simulink model "DFNN_EFS"  (R2022a)
settings: Solver=ode1  StartTime=0.0  StopTime=4*pi  FixedStep=0.001  RelTol=1e-3
libraries: roblocks x1
settings Model: Creator=DELL  LastModifiedBy=qinyi
settings DebuggingCC: UnconnectedInputMsg=warning  UnconnectedOutputMsg=warning  UnconnectedLineMsg=warning
settings RTWCC: DLArmComputeVersion=19.05

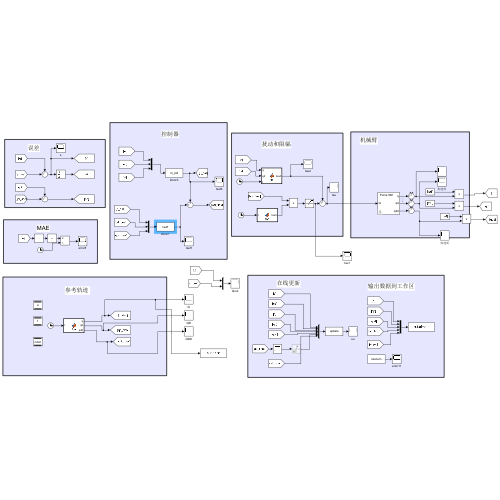
[thumbnail: Simulink's stored preview of the top-level diagram]
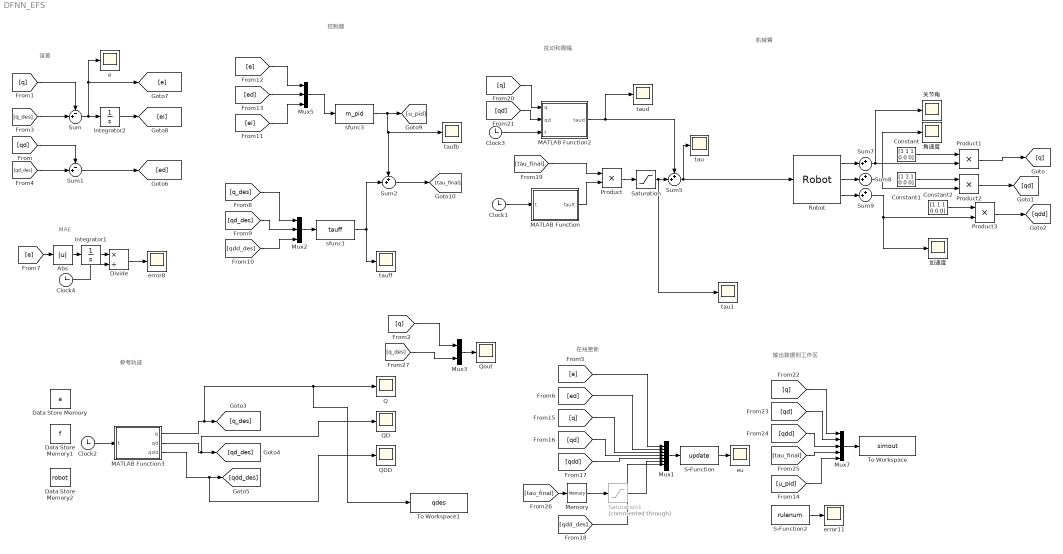
== system DFNN_EFS ==
  note: 在线更新
  note: MAE
  note: 机械臂
  note: 扰动和限幅
  note: 控制器
  note: 误差
  note: 参考轨迹
  note: 输出数据到工作区
  Abs : Abs  SaturateOnIntegerOverflow=off
  Clock{1..4} (4 alike) : Clock
  Constant : Constant  Value=[1 1 1 0 0 0]
  Constant1 : Constant  Value=[1 1 1 0 0 0]
  Constant2 : Constant  Value=[1 1 1 0 0 0]
  Data Store Memory : DataStoreMemory  DataStoreName=a  ReadBeforeWriteMsg=warning  WriteAfterWriteMsg=warning  WriteAfterReadMsg=warning  InitialValue=rand(10,6)  ShowAdditionalParam=off  OutDataTypeStr=double
  Data Store Memory1 : DataStoreMemory  DataStoreName=f  ReadBeforeWriteMsg=warning  WriteAfterWriteMsg=warning  WriteAfterReadMsg=warning  InitialValue=rand(10,6)  ShowAdditionalParam=off  OutDataTypeStr=double
  Data Store Memory2 : DataStoreMemory  DataStoreName=robot  ReadBeforeWriteMsg=warning  WriteAfterWriteMsg=warning  WriteAfterReadMsg=warning  InitialValue=rand(10,6)  ShowAdditionalParam=off  OutDataTypeStr=double
  Divide : Product  Inputs=*/
  Integrator1 : Integrator
  Integrator2 : Integrator  LimitOutput=on  UpperSaturationLimit=0.01  LowerSaturationLimit=-0.01
  MATLAB Function : MATLAB Function  TreatAsAtomicUnit=on
  MATLAB Function2 : MATLAB Function  TreatAsAtomicUnit=on
  MATLAB Function3 : MATLAB Function  TreatAsAtomicUnit=on
  Memory : Memory
  Mux1 : Mux  Inputs=7
  Mux2 : Mux  Inputs=3
  Mux3 : Mux  Inputs=2
  Mux5 : Mux  Inputs=3
  Mux7 : Mux  Inputs=5
  Product{,1..3} (4 alike) : Product
  Q : Scope
  QD : Scope
  QDD : Scope
  Qout : Scope
  Robot : roblocks/Arm/Robot  robot=p560  q0=[90 0 30 30 0 0]*pi/180
      link override Integrator: InitialCondition=0
      link override Integrator1: InitialCondition=[0 90 -90 30 0 0]'*pi/180
      link override S-Function: Parameters=p560
  S-Function : S-Function  FunctionName=update  SFunctionDeploymentMode=off  EnableBusSupport=off
  S-Function2 : S-Function  FunctionName=rulenum  SFunctionDeploymentMode=off  EnableBusSupport=off
  Saturation : Saturate  UpperLimit=800  LowerLimit=-800
  Saturation1 : Saturate  Commented=through  UpperLimit=400  LowerLimit=-400
  Sum : Sum  Inputs=-+|
  Sum1 : Sum  Inputs=-+|
  Sum{2,5,7..9} (5 alike) : Sum  Inputs=++|
  To Workspace : ToWorkspace  VariableName=simout  SaveFormat=Timeseries  SampleTime=-1
  To Workspace1 : ToWorkspace  VariableName=qdes  SaveFormat=Timeseries  SampleTime=-1
  e : Scope
  error11 : Scope
  error8 : Scope
  eu : Scope
  sfunc1 : S-Function  FunctionName=tauff  Parameters=p560  SFunctionDeploymentMode=off  EnableBusSupport=off
  sfunc3 : S-Function  FunctionName=m_pid  SFunctionDeploymentMode=off  EnableBusSupport=off
  tau : Scope
  tau1 : Scope
  taud : Scope
  taufb : Scope
  tauff : Scope
  关节角 : Scope
  加速度 : Scope
  角速度 : Scope
  wires:
  Sum/1 -> Integrator2/1, e/1, [e]
  Sum1/1 -> [ed]
  Clock1/1 -> MATLAB Function/1(t)
  Clock3/1 -> MATLAB Function2/3(t)
  Mux2/1 -> sfunc1/1
  Sum5/1 -> Robot/1, tau/1
  Abs/1 -> Integrator1/1
  Integrator1/1 -> Divide/1
  Divide/1 -> error8/1
  Mux5/1 -> sfunc3/1
  S-Function/1 -> eu/1
  Mux7/1 -> To Workspace/1
  S-Function2/1 -> error11/1
  sfunc1/1 -> Sum2/2, tauff/1
  Mux1/1 -> S-Function/1
  Sum7/1 -> Product1/2, 关节角/1
  Sum8/1 -> 角速度/1, Product2/2
  Sum9/1 -> Product3/2, 加速度/1
  Integrator2/1 -> [ei]
  MATLAB Function/1(fault) -> Product/2
  Clock2/1 -> MATLAB Function3/1(t)
  MATLAB Function3/1(q) -> To Workspace1/1, Q/1, [q_des]
  MATLAB Function3/2(qd) -> QD/1, [qd_des]
  MATLAB Function3/3(qdd) -> QDD/1, [qdd_des]
  Clock4/1 -> Divide/2
  [q] -> Sum/1
  [qd] -> Sum1/1
  [q_des] -> Sum/2
  [qd_des] -> Sum1/2
  [e] -> Mux1/1
  [ed] -> Mux1/2
  [e] -> Abs/1
  [q_des] -> Mux2/1
  [qd_des] -> Mux2/2
  [qdd_des] -> Mux2/3
  [e] -> Mux5/1
  [ed] -> Mux5/2
  [ei] -> Mux5/3
  sfunc3/1 -> taufb/1, Sum2/1, [u_pid]
  [u_pid] -> Mux7/5
  [q] -> Mux1/3
  [qd] -> Mux1/4
  [qdd] -> Mux1/5
  [qdd_des] -> Mux1/7
  Sum2/1 -> [tau_final]
  [tau_final] -> Product/1
  [q] -> MATLAB Function2/1(q)
  [qd] -> MATLAB Function2/2(qd)
  MATLAB Function2/1(taud) -> taud/1, Sum5/1
  Robot/1 -> Sum7/2
  Robot/2 -> Sum8/2
  Robot/3 -> Sum9/2
  [q] -> Mux7/1
  [qd] -> Mux7/2
  [qdd] -> Mux7/3
  [tau_final] -> Mux7/4
  [tau_final] -> Memory/1
  Product/1 -> Saturation/1
  Saturation/1 -> tau1/1, Sum5/2
  Constant/1 -> Product1/1
  Product2/1 -> [qd]
  Product3/1 -> [qdd]
  Constant1/1 -> Product2/1
  Constant2/1 -> Product3/1
  Product1/1 -> [q]
  Mux3/1 -> Qout/1
  [q] -> Mux3/1
  [q_des] -> Mux3/2
  Memory/1 -> Saturation1/1
  Saturation1/1 -> Mux1/6

== matlab function DFNN_EFS/MATLAB Function2 ==
  settings: updateMethod=DISCRETE
  data: q input; qd input; t input; taud output; a data_store_memory; f data_store_memory
function taud  = dis(q,qd,t)
rng(1);
taud=[30; 30 ;30 ;10 ;10 ;10]*sin(0.3*pi*t)+[5; 5 ;5 ;5 ;5 ;5].*sin(q).*qd+[1; 1; 1; 1; 1; 1].*qd+randn(6,1);
%     taud=taud*(1-exp(-0.3*(t-10)));
%     taud=[50; 50 ;50 ;15 ;15 ;15];
taud=1*taud;
if(t<2*pi)
    taud=0*taud;
else

end

== matlab function DFNN_EFS/MATLAB Function ==
  data: t input; fault output
 function fault = fcn(t)
if(t>2*pi)
    fault = 0.5+0.5*exp(-0.3*(t-2*pi));
else
    fault=1;
end

== matlab function DFNN_EFS/MATLAB Function3 ==
  settings: updateMethod=DISCRETE
  data: t input; q output; qd output; qdd output; a data_store_memory; f data_store_memory
function [q,qd,qdd] = fcn(t)

% if(t >= 2*pi && t < 4*pi)
%     B=[80 70 70 0 0 0]*pi/180;
%     q = [0.4*B.*sign(sin(ones(1,6)*2*t))]'+[0 90 -90 0 0 0]'*pi/180;
%     qd = ones(6,1);
%     qdd = ones(6,1);
% else
%     fq=1*ones(1,6);
%     B=[80 70 70 0 0 0]*pi/180;
%     q=[B.*sin(fq*t)]'+[0 90 -90 0 0 0]'*pi/180;
%     qd=[B.*fq.*cos(fq*t)]';
%     qdd=[-B.*fq.*fq.*sin(fq*t)]';
% end

deg2rad = pi/180;

% 参数
h1 = 80 * deg2rad;       % 位置梯形高度
h2 = 70 * deg2rad;
h3 = 70 * deg2rad;
T = pi;                 % 总时间
t_top = 4 * pi / 6;     % 顶部保持段长度
t_side = (T - t_top);   % 两侧斜边时间总和
t_rise = t_side / 2;    % 上升时间
t_fall = t_rise;        % 下降时间

% 匀速速度
v_const1 = h1 / t_rise;
v_const2 = h2 / t_rise;
v_const3 = h3 / t_rise;

if(t >= 2*pi&& t < 3*pi)
    if t < t_rise+2*pi
        % 位置匀速上升
        q1 = v_const1 * (t-2*pi);
        q2 = v_const2 * (t-2*pi);
        q3 = v_const3 * (t-2*pi);
        qd1 = v_const1;
        qd2 = v_const1;
        qd3 = v_const1;
        qdd = zeros(6,1);
        q=[q1 q2 q3 0 0 0]'+ +[0 90 -90 0 0 0]'*pi/180;
        qd = [qd1 qd2 qd3 0 0 0]';
    elseif t < t_rise + t_top + 2*pi
        % 匀速段
        q1 = h1;
        q2 = h2;
        q3 = h3;
        qdd = zeros(6,1);
        q=[q1 q2 q3 0 0 0]'+ +[0 90 -90 0 0 0]'*pi/180;
        qd = [0 0 0 0 0 0]';
    else
        % 减速段
        q1 = h1 - v_const1 * (t - t_rise - t_top-2*pi);
        q2 = h2 - v_const2 * (t - t_rise - t_top-2*pi);
        q3 = h3 - v_const3 * (t - t_rise - t_top-2*pi);
        qd1 = -v_const1;
        qd2 = -v_const2;
        qd3 = -v_const3;
        qdd = zeros(6,1);
        q=[q1 q2 q3 0 0 0]'+ +[0 90 -90 0 0 0]'*pi/180;
        qd = [qd1 qd2 qd3 0 0 0]';
    end
elseif(t >= 3*pi)
    if t < t_rise+3*pi
        % 位置匀速上升
        q1 = -v_const1 * (t-3*pi);
        q2 = -v_const2 * (t-3*pi);
        q3 = -v_const3 * (t-3*pi);
        qd1 = -v_const1;
        qd2 = -v_const2;
        qd3 = -v_const3;
        qdd = zeros(6,1);
        q=[q1 q2 q3 0 0 0]'+ +[0 90 -90 0 0 0]'*pi/180;
        qd = [qd1 qd2 qd3 0 0 0]';
    elseif t < t_rise + t_top + 3*pi
        % 匀速段
        q1 = -h1;
        q2 = -h2;
        q3 = -h3;
        qdd = zeros(6,1);
        q=[q1 q2 q3 0 0 0]'+ +[0 90 -90 0 0 0]'*pi/180;
        qd = [0 0 0 0 0 0]';
    else
        % 减速段
        q1 = -h1 + v_const1 * (t - t_rise - t_top-3*pi);
        q2 = -h2 + v_const1 * (t - t_rise - t_top-3*pi);
        q3 = -h3 + v_const1 * (t - t_rise - t_top-3*pi);
        qd1 = v_const1;
        qd2 = v_const2;
        qd3 = v_const3;
        qdd = zeros(6,1);
        q=[q1 q2 q3 0 0 0]'+ +[0 90 -90 0 0 0]'*pi/180;
        qd = [qd1 qd2 qd3 0 0 0]';
    end

else
    fq=1*ones(1,6);
    B=[80 70 70 0 0 0]*pi/180;
    q=[B.*sin(fq*t)]'+[0 90 -90 0 0 0]'*pi/180;
    qd=[B.*fq.*cos(fq*t)]';
    qdd=[-B.*fq.*fq.*sin(fq*t)]';
end
